simulink model "FaultDetection"  (R2023a)
settings: configuration reference "AutosarConfig" (kept outside this file)
values from neighbouring files (symbols this model uses):
  Contact : value not decoded    [BMS_Software_DD.sldd]
  HighCellTempLimit = 55.0    [BMS_Software_DD.sldd]
  LowCellTempLimit = -15.0    [BMS_Software_DD.sldd]
  OverCellVoltageLimit = 4.25    [BMS_Software_DD.sldd]
  UnderCellVoltageLimit = 2.5    [BMS_Software_DD.sldd]
libraries: BatteryProtection x8, simulink x7
settings Model: DataDictionary=BMS_Software_DD.sldd  EnableAccessToBaseWorkspace=off  Creator=cpatel  LastModifiedBy=cpatel
settings ConfigSetRef: SourceName=AutosarConfig

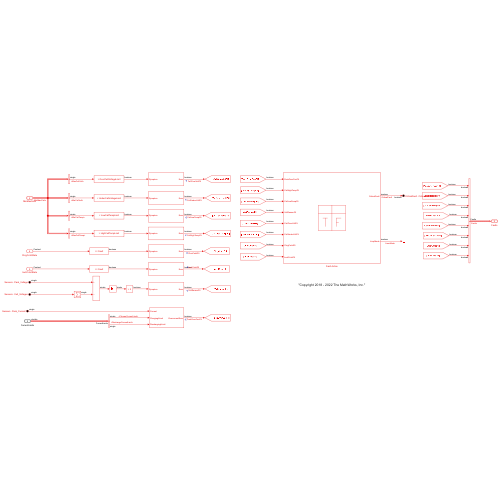
[thumbnail: Simulink's stored preview of the top-level diagram]
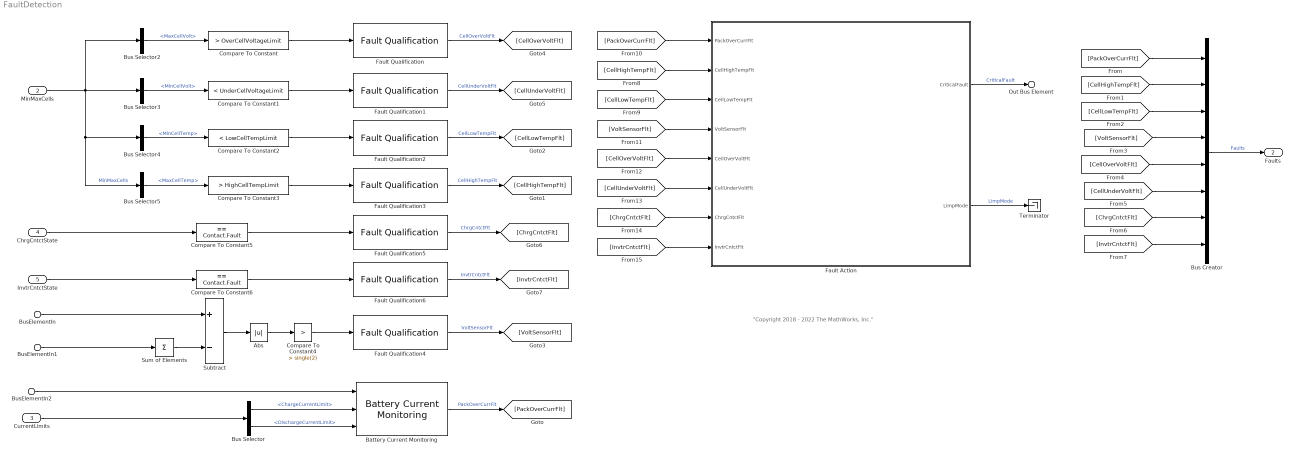
== system FaultDetection ==
  note: "Copyright 2018 - 2022 The MathWorks, Inc."
  BusElementIn1 : Inport  PortName=Sensors  Element=Cell_Voltages
  BusElementIn : Inport  PortName=Sensors  Element=Pack_Voltage
  BusElementIn2 : Inport  PortName=Sensors  Element=Pack_Current
  MinMaxCells : Inport  Port=2  OutDataTypeStr=Bus: Min_Max_Cells
  CurrentLimits : Inport  Port=3  OutDataTypeStr=Bus: CurrentLimits
  ChrgCntctState : Inport  Port=4  OutDataTypeStr=Enum: Contact
  InvtrCntctState : Inport  Port=5  OutDataTypeStr=Enum: Contact
  Abs : Abs  SaturateOnIntegerOverflow=off
  Battery Current Monitoring : BatteryProtection/Battery Current Monitoring  ErrorLimit=0  QualTime=2  DisqualTime=4  Ts=0.1
      settings: LibrarySourceBlock=|
      | batt_sl_lib/Protection/Battery Current
      | Monitoring
  Bus Creator : BusCreator  Inputs=8  OutDataTypeStr=Bus: Faults  NonVirtualBus=on
      settings: InheritFromInputs=off
  Bus Selector : BusSelector  OutputSignals=ChargeCurrentLimit,DischargeCurrentLimit
  Bus Selector2 : BusSelector  OutputSignals=MaxCellVolt
  Bus Selector3 : BusSelector  OutputSignals=MinCellVolt
  Bus Selector4 : BusSelector  OutputSignals=MinCellTemp
  Bus Selector5 : BusSelector  OutputSignals=MaxCellTemp
  Compare To Constant : simulink/Logic and Bit Operations/Compare To Constant  relop=>  const=OverCellVoltageLimit  OutDataTypeStr=boolean
  Compare To Constant1 : simulink/Logic and Bit Operations/Compare To Constant  relop=<  const=UnderCellVoltageLimit  OutDataTypeStr=boolean
  Compare To Constant2 : simulink/Logic and Bit Operations/Compare To Constant  relop=<  const=LowCellTempLimit  OutDataTypeStr=boolean
  Compare To Constant3 : simulink/Logic and Bit Operations/Compare To Constant  relop=>  const=HighCellTempLimit  OutDataTypeStr=boolean
  Compare To Constant4 : simulink/Logic and Bit Operations/Compare To Constant  relop=>  const=single(2)  OutDataTypeStr=boolean
  Compare To Constant5 : simulink/Logic and Bit Operations/Compare To Constant  relop===  const=Contact.Fault  OutDataTypeStr=boolean
  Compare To Constant6 : simulink/Logic and Bit Operations/Compare To Constant  relop===  const=Contact.Fault  OutDataTypeStr=boolean
  Fault Action : Truth Table  TreatAsAtomicUnit=on
  Fault Qualification : BatteryProtection/Fault Qualification  QualTime=2  DisqualTime=4  Ts=0.1
      settings: LibrarySourceBlock=batt_sl_lib/Protection/Fault Qualification
  Fault Qualification1 : BatteryProtection/Fault Qualification  QualTime=2  DisqualTime=4  Ts=0.1
      settings: LibrarySourceBlock=batt_sl_lib/Protection/Fault Qualification
  Fault Qualification2 : BatteryProtection/Fault Qualification  QualTime=4  DisqualTime=6  Ts=0.1
      settings: LibrarySourceBlock=batt_sl_lib/Protection/Fault Qualification
  Fault Qualification3 : BatteryProtection/Fault Qualification  QualTime=4  DisqualTime=6  Ts=0.1
      settings: LibrarySourceBlock=batt_sl_lib/Protection/Fault Qualification
  Fault Qualification4 : BatteryProtection/Fault Qualification  QualTime=2  DisqualTime=4  Ts=0.1
      settings: LibrarySourceBlock=batt_sl_lib/Protection/Fault Qualification
  Fault Qualification5 : BatteryProtection/Fault Qualification  QualTime=0.5  DisqualTime=2  Ts=0.1
      settings: LibrarySourceBlock=batt_sl_lib/Protection/Fault Qualification
  Fault Qualification6 : BatteryProtection/Fault Qualification  QualTime=0.5  DisqualTime=2  Ts=0.1
      settings: LibrarySourceBlock=batt_sl_lib/Protection/Fault Qualification
  Subtract : Sum  Inputs=+-
  Sum of Elements : Sum  Inputs=+
  Terminator : Terminator
  Out Bus Element : Outport  PortName=CriticalFault  Element=CriticalFault
  Faults : Outport  Port=2  OutDataTypeStr=Bus: Faults
  wires:
  Fault Action/2(LimpMode) -> Terminator/1  "LimpMode"
  Fault Qualification5/1 -> [ChrgCntctFlt]  "ChrgCntctFlt"
  Fault Qualification6/1 -> [InvtrCntctFlt]  "InvtrCntctFlt"
  [PackOverCurrFlt] -> Fault Action/1(PackOverCurrFlt)
  [PackOverCurrFlt] -> Bus Creator/1
  [CellHighTempFlt] -> Bus Creator/2
  [CellLowTempFlt] -> Bus Creator/3
  [VoltSensorFlt] -> Bus Creator/4
  [CellOverVoltFlt] -> Bus Creator/5
  [CellUnderVoltFlt] -> Bus Creator/6
  [ChrgCntctFlt] -> Bus Creator/7
  [InvtrCntctFlt] -> Bus Creator/8
  [CellHighTempFlt] -> Fault Action/2(CellHighTempFlt)
  [CellLowTempFlt] -> Fault Action/3(CellLowTempFlt)
  [VoltSensorFlt] -> Fault Action/4(VoltSensorFlt)
  [CellOverVoltFlt] -> Fault Action/5(CellOverVoltFlt)
  [CellUnderVoltFlt] -> Fault Action/6(CellUnderVoltFlt)
  [ChrgCntctFlt] -> Fault Action/7(ChrgCntctFlt)
  [InvtrCntctFlt] -> Fault Action/8(InvtrCntctFlt)
  Fault Qualification/1 -> [CellOverVoltFlt]  "CellOverVoltFlt"
  Compare To Constant2/1 -> Fault Qualification2/1
  Fault Qualification4/1 -> [VoltSensorFlt]  "VoltSensorFlt"
  Compare To Constant4/1 -> Fault Qualification4/1
  Compare To Constant1/1 -> Fault Qualification1/1
  Fault Qualification1/1 -> [CellUnderVoltFlt]  "CellUnderVoltFlt"
  Compare To Constant3/1 -> Fault Qualification3/1
  Fault Qualification2/1 -> [CellLowTempFlt]  "CellLowTempFlt"
  Compare To Constant/1 -> Fault Qualification/1
  BusElementIn1/1 -> Sum of Elements/1
  Bus Selector5/1 -> Compare To Constant3/1  "<MaxCellTemp>"
  Bus Selector3/1 -> Compare To Constant1/1  "<MinCellVolt>"
  Bus Selector2/1 -> Compare To Constant/1  "<MaxCellVolt>"
  Abs/1 -> Compare To Constant4/1
  Subtract/1 -> Abs/1
  Fault Qualification3/1 -> [CellHighTempFlt]  "CellHighTempFlt"
  Bus Selector4/1 -> Compare To Constant2/1  "<MinCellTemp>"
  Sum of Elements/1 -> Subtract/2
  BusElementIn/1 -> Subtract/1
  BusElementIn2/1 -> Battery Current Monitoring/1
  Bus Selector/1 -> Battery Current Monitoring/2  "<ChargeCurrentLimit>"
  Bus Selector/2 -> Battery Current Monitoring/3  "<DischargeCurrentLimit>"
  Battery Current Monitoring/1 -> [PackOverCurrFlt]  "PackOverCurrFlt"
  Compare To Constant5/1 -> Fault Qualification5/1
  Compare To Constant6/1 -> Fault Qualification6/1
  Fault Action/1(CriticalFault) -> Out Bus Element/1  "CriticalFault"
  Bus Creator/1 -> Faults/1  "Faults"
  ChrgCntctState/1 -> Compare To Constant5/1
  CurrentLimits/1 -> Bus Selector/1
  InvtrCntctState/1 -> Compare To Constant6/1
  MinMaxCells/1 -> Bus Selector5/1, Bus Selector4/1, Bus Selector3/1, Bus Selector2/1  "MinMaxCells"

== matlab function FaultDetection/Fault Action ==
  data: PackOverCurrFlt input; CriticalFault output boolean size=1 =false; CellHighTempFlt input; CellLowTempFlt input; VoltSensorFlt input; CellOverVoltFlt input; CellUnderVoltFlt input; ChrgCntctFlt input; InvtrCntctFlt input; LimpMode output boolean =false
function [CriticalFault, LimpMode] = fcn(PackOverCurrFlt, CellHighTempFlt, CellLowTempFlt, VoltSensorFlt, CellOverVoltFlt, CellUnderVoltFlt, ChrgCntctFlt, InvtrCntctFlt)

aVarTruthTableCondition_1 = false;
aVarTruthTableCondition_2 = false;


% Any Non-Critical Fault Active

aVarTruthTableCondition_1 = logical(PackOverCurrFlt || CellHighTempFlt || CellLowTempFlt || CellOverVoltFlt || CellUnderVoltFlt ||   VoltSensorFlt);

% Critical Fault Active

aVarTruthTableCondition_2 = logical(ChrgCntctFlt || InvtrCntctFlt);

if (aVarTruthTableCondition_1)
    aFcnTruthTableAction_3();
elseif (aVarTruthTableCondition_2)
    aFcnTruthTableAction_2();
else % Default
    aFcnTruthTableAction_1();
end

function aFcnTruthTableAction_1()

% No Fault Not Present

CriticalFault = false;
LimpMode = false;

function aFcnTruthTableAction_2()

% Critical Fault Present

CriticalFault = true;

function aFcnTruthTableAction_3()

% Limp Mode Active

LimpMode = true;
